simulink model "project_3_Matrixop"  (R2023a)
settings: Solver=VariableStepAuto  StartTime=0.0  StopTime=10  RelTol=1e-3
values from neighbouring files (symbols this model uses):
  m1 = input('ENTER 1ST MAT')    [project_3_Matrixop_script.m]
  m2 = input('ENTER 2ND MAT')    [project_3_Matrixop_script.m]
settings Model: Creator=FC  LastModifiedBy=FC

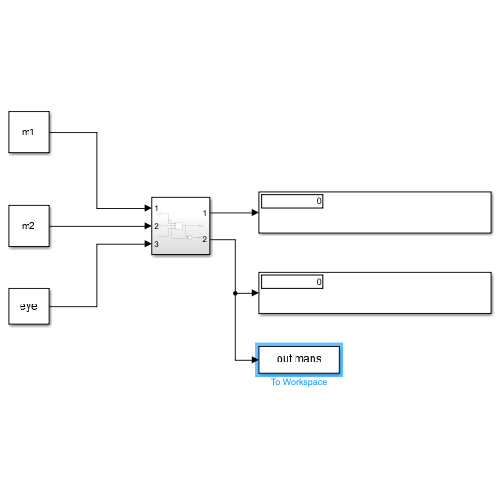
[thumbnail: Simulink's stored preview of the top-level diagram]
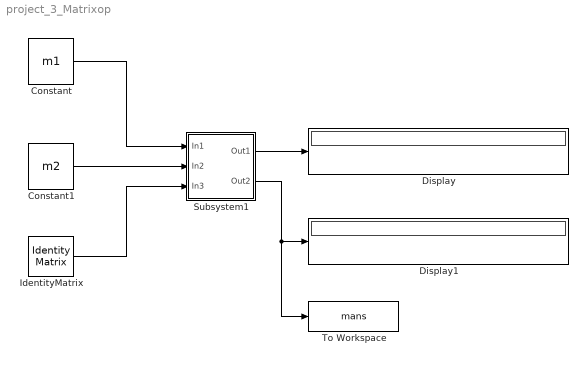
== system project_3_Matrixop ==
  Constant : Constant  Value=m1  VectorParams1D=off
  Constant1 : Constant  Value=m2  VectorParams1D=off
  Display : Display
  Display1 : Display
  IdentityMatrix : IdentityMatrix  OutputDimensions=m3
  Subsystem1 : Subsystem
  To Workspace : ToWorkspace  VariableName=mans
      settings: Save2DSignal=2-D array (concatenate along first dimension)
  wires:
  Constant/1 -> Subsystem1/1(In1)
  Constant1/1 -> Subsystem1/2(In2)
  IdentityMatrix/1 -> Subsystem1/3(In3)
  Subsystem1/1(Out1) -> Display/1
  Subsystem1/2(Out2) -> To Workspace/1, Display1/1

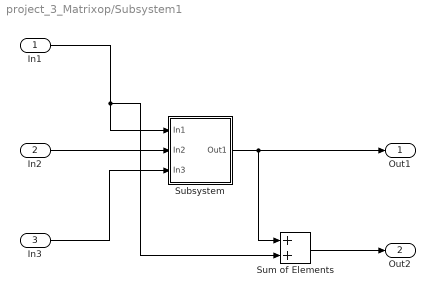
== system project_3_Matrixop/Subsystem1 ==
  In1 : Inport
  In2 : Inport  Port=2
  In3 : Inport  Port=3
  Subsystem : Subsystem
  Sum of Elements : Sum
  Out1 : Outport
  Out2 : Outport  Port=2
  wires:
  In3/1 -> Subsystem/3(In3)
  In1/1 -> Sum of Elements/2, Subsystem/1(In1)
  Sum of Elements/1 -> Out2/1
  Subsystem/1(Out1) -> Out1/1, Sum of Elements/1
  In2/1 -> Subsystem/2(In2)

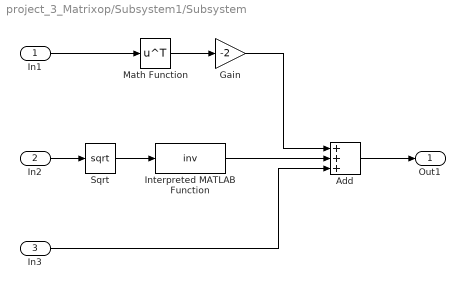
== system project_3_Matrixop/Subsystem1/Subsystem ==
  In1 : Inport
  In2 : Inport  Port=2
  In3 : Inport  Port=3
  Add : Sum  Inputs=+++
  Gain : Gain  Gain=-2
  Interpreted MATLAB Function : MATLABFcn  MATLABFcn=inv  Output1D=off
  Math Function : Math  Operator=transpose
  Sqrt : Sqrt
  Out1 : Outport
  wires:
  Interpreted MATLAB Function/1 -> Add/2
  Add/1 -> Out1/1
  Gain/1 -> Add/1
  In1/1 -> Math Function/1
  In2/1 -> Sqrt/1
  Sqrt/1 -> Interpreted MATLAB Function/1
  Math Function/1 -> Gain/1
  In3/1 -> Add/3
